simulink model "ModeAdjust"  (R2018b)
(part 6 of 35)

  PA_KeSMSw4sLyingMDSecRwRtStLgrstOtwdInwdPosMax_Val/1 -> Bus Creator74/11  "LgrstOtwdInwdPosMax"
  PA_KeSMSw4sLyingMDSecRwRtStBkReclnUpwdDnwdPosMax_Val/1 -> Bus Creator74/2  "BkReclnUpwdDnwdPosMax"
  PA_KeSMSw4sLyingMDSecRwRtStLgrstUpwdPosMin_Val/1 -> Bus Creator74/9  "LgrstUpwdPosMin"
  PA_KeSMSw4sLyingMDSecRwRtStLgrstUpwdPosMax_Val/1 -> Bus Creator74/8  "LgrstUpwdPosMax"
  PA_KeSMSw4sLyingMDSecRwRtStHdrstUpwdPosMin_Val/1 -> Bus Creator74/6  "HdrstUpwdPosMin"
  PA_KeSMSw4sLyingMDSecRwRtStFtrstUpwdDnwdPosMax_Val/1 -> Bus Creator74/14  "FtrstUpwdDnwdPosMax"
  PA_KeSMSw4sLyingMDSecRwRtStFtrstUpwdDnwdPosMin_Val/1 -> Bus Creator74/15  "FtrstUpwdDnwdPosMin"
  PA_KeSMSw4sLyingMDSecRwRtStBkReclnUpwdDnwdPos_Val/1 -> Bus Creator74/1  "BkReclnUpwdDnwdPos"
  PA_KeSMSw4sLyingMDSecRwRtStHdrstUpwdPos_Val/1 -> Bus Creator74/4  "HdrstUpwdPos"
  PA_KeSMSw4sLyingMDSecRwRtStHdrstUpwdPosMax_Val/1 -> Bus Creator74/5  "HdrstUpwdPosMax"
  PA_KeSMSw4sLyingMDSecRwRtStFtrstUpwdDnwdPos_Val/1 -> Bus Creator74/13  "FtrstUpwdDnwdPos"
  PA_KeSMSw4sRecoveryMDSecRwLtStFtrstUpwdDnwdPos_Val/1 -> Bus Creator75/13  "FtrstUpwdDnwdPos"
  PA_KeSMSw4sRecoveryMDSecRwLtStFtrstUpwdDnwdPosMin_Val/1 -> Bus Creator75/15  "FtrstUpwdDnwdPosMin"
  PA_KeSMSw4sRecoveryMDSecRwLtStFtrstUpwdDnwdPosMax_Val/1 -> Bus Creator75/14  "FtrstUpwdDnwdPosMax"
  PA_KeSMSw4sRecoveryMDSecRwLtStLgrstOtwdInwdPos_Val/1 -> Bus Creator75/10  "LgrstOtwdInwdPos"
  PA_KeSMSw4sRecoveryMDSecRwLtStLgrstOtwdInwdPosMin_Val/1 -> Bus Creator75/12  "LgrstOtwdInwdPosMin"
  PA_KeSMSw4sRecoveryMDSecRwLtStLgrstOtwdInwdPosMax_Val/1 -> Bus Creator75/11  "LgrstOtwdInwdPosMax"
  PA_KeSMSw4sRecoveryMDSecRwLtStLgrstUpwdDnwdPosMin_Val/1 -> Bus Creator75/9  "LgrstUpwdPosMin"
  PA_KeSMSw4sRecoveryMDSecRwLtStHdrstUpwdDnwdPosMax_Val/1 -> Bus Creator75/5  "HdrstUpwdPosMax"
  PA_KeSMSw4sRecoveryMDSecRwLtStBkReclnUpwdDnwdPosMax_Val/1 -> Bus Creator75/2  "BkReclnUpwdDnwdPosMax"
  PA_KeSMSw4sRecoveryMDSecRwLtStBkReclnUpwdDnwdPos_Val/1 -> Bus Creator75/1  "BkReclnUpwdDnwdPos"
  PA_KeSMSw4sRecoveryMDSecRwLtStHdrstUpwdDnwdPos_Val/1 -> Bus Creator75/4  "HdrstUpwdPos"
  PA_KeSMSw4sRecoveryMDSecRwLtStLgrstUpwdDnwdPosMax_Val/1 -> Bus Creator75/8  "LgrstUpwdPosMax"
  PA_KeSMSw4sRecoveryMDSecRwLtStLgrstUpwdDnwdPos_Val/1 -> Bus Creator75/7  "LgrstUpwdPos"
  PA_KeSMSw4sRecoveryMDSecRwLtStHdrstUpwdDnwdPosMin_Val/1 -> Bus Creator75/6  "HdrstUpwdPosMin"
  PA_KeSMSw4sRecoveryMDSecRwLtStBkReclnUpwdDnwdPosMin_Val/1 -> Bus Creator75/3  "BkReclnUpwdDnwdPosMin"
  PA_KeSMSw4sRecoveryMDSecRwRtStFtrstUpwdDnwdPos_Val/1 -> Bus Creator76/13  "FtrstUpwdDnwdPos"
  PA_KeSMSw4sRecoveryMDSecRwRtStHdrstUpwdPosMax_Val/1 -> Bus Creator76/5  "HdrstUpwdPosMax"
  PA_KeSMSw4sRecoveryMDSecRwRtStHdrstUpwdPos_Val/1 -> Bus Creator76/4  "HdrstUpwdPos"
  PA_KeSMSw4sRecoveryMDSecRwRtStBkReclnUpwdDnwdPos_Val/1 -> Bus Creator76/1  "BkReclnUpwdDnwdPos"
  PA_KeSMSw4sRecoveryMDSecRwRtStFtrstUpwdDnwdPosMin_Val/1 -> Bus Creator76/15  "FtrstUpwdDnwdPosMin"
  PA_KeSMSw4sRecoveryMDSecRwRtStFtrstUpwdDnwdPosMax_Val/1 -> Bus Creator76/14  "FtrstUpwdDnwdPosMax"
  PA_KeSMSw4sRecoveryMDSecRwRtStHdrstUpwdPosMin_Val/1 -> Bus Creator76/6  "HdrstUpwdPosMin"
  PA_KeSMSw4sRecoveryMDSecRwRtStLgrstUpwdPosMax_Val/1 -> Bus Creator76/8  "LgrstUpwdPosMax"
  PA_KeSMSw4sRecoveryMDSecRwRtStLgrstUpwdPosMin_Val/1 -> Bus Creator76/9  "LgrstUpwdPosMin"
  PA_KeSMSw4sRecoveryMDSecRwRtStBkReclnUpwdDnwdPosMax_Val/1 -> Bus Creator76/2  "BkReclnUpwdDnwdPosMax"
  PA_KeSMSw4sRecoveryMDSecRwRtStLgrstOtwdInwdPosMax_Val/1 -> Bus Creator76/11  "LgrstOtwdInwdPosMax"
  PA_KeSMSw4sRecoveryMDSecRwRtStBkReclnUpwdDnwdPosMin_Val/1 -> Bus Creator76/3  "BkReclnUpwdDnwdPosMin"
  PA_KeSMSw4sRecoveryMDSecRwRtStLgrstOtwdInwdPosMin_Val/1 -> Bus Creator76/12  "LgrstOtwdInwdPosMin"
  PA_KeSMSw4sRecoveryMDSecRwRtStLgrstOtwdInwdPos_Val/1 -> Bus Creator76/10  "LgrstOtwdInwdPos"
  PA_KeSMSw4sRecoveryMDSecRwRtStLgrstUpwdPos_Val/1 -> Bus Creator76/7  "LgrstUpwdPos"
  PA_KeSMSw4sVIPMDSecRwLtStBkReclnUpwdDnwdPosMin_Val/1 -> Bus Creator77/3  "BkReclnUpwdDnwdPosMin"
  PA_KeSMSw4sVIPMDSecRwLtStHdrstUpwdDnwdPosMin_Val/1 -> Bus Creator77/6  "HdrstUpwdPosMin"
  PA_KeSMSw4sVIPMDSecRwLtStLgrstUpwdDnwdPos_Val/1 -> Bus Creator77/7  "LgrstUpwdPos"
  PA_KeSMSw4sVIPMDSecRwLtStLgrstUpwdDnwdPosMax_Val/1 -> Bus Creator77/8  "LgrstUpwdPosMax"
  PA_KeSMSw4sVIPMDSecRwLtStHdrstUpwdDnwdPos_Val/1 -> Bus Creator77/4  "HdrstUpwdPos"
  PA_KeSMSw4sVIPMDSecRwLtStBkReclnUpwdDnwdPos_Val/1 -> Bus Creator77/1  "BkReclnUpwdDnwdPos"
  PA_KeSMSw4sVIPMDSecRwLtStBkReclnUpwdDnwdPosMax_Val/1 -> Bus Creator77/2  "BkReclnUpwdDnwdPosMax"
  PA_KeSMSw4sVIPMDSecRwLtStHdrstUpwdDnwdPosMax_Val/1 -> Bus Creator77/5  "HdrstUpwdPosMax"
  PA_KeSMSw4sVIPMDSecRwLtStLgrstUpwdDnwdPosMin_Val/1 -> Bus Creator77/9  "LgrstUpwdPosMin"
  PA_KeSMSw4sVIPMDSecRwLtStLgrstOtwdInwdPosMax_Val/1 -> Bus Creator77/11  "LgrstOtwdInwdPosMax"
  PA_KeSMSw4sVIPMDSecRwLtStLgrstOtwdInwdPosMin_Val/1 -> Bus Creator77/12  "LgrstOtwdInwdPosMin"
  PA_KeSMSw4sVIPMDSecRwLtStLgrstOtwdInwdPos_Val/1 -> Bus Creator77/10  "LgrstOtwdInwdPos"
  PA_KeSMSw4sVIPMDSecRwLtStFtrstUpwdDnwdPosMax_Val/1 -> Bus Creator77/14  "FtrstUpwdDnwdPosMax"
  PA_KeSMSw4sVIPMDSecRwLtStFtrstUpwdDnwdPosMin_Val/1 -> Bus Creator77/15  "FtrstUpwdDnwdPosMin"
  PA_KeSMSw4sVIPMDSecRwLtStFtrstUpwdDnwdPos_Val/1 -> Bus Creator77/13  "FtrstUpwdDnwdPos"
  PA_KeSMSw4sVIPMDSecRwRtStLgrstUpwdPos_Val/1 -> Bus Creator78/7  "LgrstUpwdPos"
  PA_KeSMSw4sVIPMDSecRwRtStLgrstOtwdInwdPos_Val/1 -> Bus Creator78/10  "LgrstOtwdInwdPos"
  PA_KeSMSw4sVIPMDSecRwRtStLgrstOtwdInwdPosMin_Val/1 -> Bus Creator78/12  "LgrstOtwdInwdPosMin"
  PA_KeSMSw4sVIPMDSecRwRtStBkReclnUpwdDnwdPosMin_Val/1 -> Bus Creator78/3  "BkReclnUpwdDnwdPosMin"
  PA_KeSMSw4sVIPMDSecRwRtStLgrstOtwdInwdPosMax_Val/1 -> Bus Creator78/11  "LgrstOtwdInwdPosMax"
  PA_KeSMSw4sVIPMDSecRwRtStBkReclnUpwdDnwdPosMax_Val/1 -> Bus Creator78/2  "BkReclnUpwdDnwdPosMax"
  PA_KeSMSw4sVIPMDSecRwRtStLgrstUpwdPosMin_Val/1 -> Bus Creator78/9  "LgrstUpwdPosMin"
  PA_KeSMSw4sVIPMDSecRwRtStLgrstUpwdPosMax_Val/1 -> Bus Creator78/8  "LgrstUpwdPosMax"
  PA_KeSMSw4sVIPMDSecRwRtStHdrstUpwdPosMin_Val/1 -> Bus Creator78/6  "HdrstUpwdPosMin"
  PA_KeSMSw4sVIPMDSecRwRtStFtrstUpwdDnwdPosMax_Val/1 -> Bus Creator78/14  "FtrstUpwdDnwdPosMax"
  PA_KeSMSw4sVIPMDSecRwRtStFtrstUpwdDnwdPosMin_Val/1 -> Bus Creator78/15  "FtrstUpwdDnwdPosMin"
  PA_KeSMSw4sVIPMDSecRwRtStBkReclnUpwdDnwdPos_Val/1 -> Bus Creator78/1  "BkReclnUpwdDnwdPos"
  PA_KeSMSw4sVIPMDSecRwRtStHdrstUpwdPos_Val/1 -> Bus Creator78/4  "HdrstUpwdPos"
  PA_KeSMSw4sVIPMDSecRwRtStHdrstUpwdPosMax_Val/1 -> Bus Creator78/5  "HdrstUpwdPosMax"
  PA_KeSMSw4sVIPMDSecRwRtStFtrstUpwdDnwdPos_Val/1 -> Bus Creator78/13  "FtrstUpwdDnwdPos"
  Bus Creator75/1 -> Bus Creator79/2  "RecvyLSecRwLtSt"
  Bus Creator77/1 -> Bus Creator79/3  "VipLSecRwLtSt"
  Bus Creator73/1 -> Bus Creator79/1  "LyLSecRwLtSt"
  Bus Creator76/1 -> Bus Creator80/2  "RecvyRSecRwRtSt"
  Bus Creator74/1 -> Bus Creator80/1  "LyRSecRwRtSt"
  Bus Creator78/1 -> Bus Creator80/3  "VipRSecRwRtSt"
  Bus Creator79/1 -> [Calib_2L4s]
  Bus Creator80/1 -> [Calib_2R4s]
  [Calib_2L4s] -> Bus Creator26/7  "Calib_2L4s"
  [Calib_2R4s] -> Bus Creator26/8  "Calib_2R4s"
  PA_KeSMSw6sRecoveryDrvStFtUpwdDnwdPosMax_Val/1 -> Bus Creator81/8  "FtUpwdDnwdPosMax"
  PA_KeSMSwDltTrgtPos_Val23/1 -> Bus Creator81/4  "FrwdBkwdPos"
  PA_KeSMSw6sRecoveryDrvStFtUpwdDnwdPosMin_Val/1 -> Bus Creator81/9  "FtUpwdDnwdPosMin"
  PA_KeSMSwDltTrgtPos_Val20/1 -> Bus Creator81/1  "BkReclnUpwdDnwdPos"
  PA_KeSMSwDltTrgtPos_Val22/1 -> Bus Creator81/5  "FrwdBkwdPosMax"
  PA_KeSMSwDltTrgtPos_Val19/1 -> Bus Creator81/2  "BkReclnUpwdDnwdPosMax"
  PA_KeSMSw6sRecoveryDrvStFtUpwdDnwdPos_Val/1 -> Bus Creator81/7  "FtUpwdDnwdPos"
  PA_KeSMSwDltTrgtPos_Val24/1 -> Bus Creator81/6  "FrwdBkwdPosMin"
  Bus Creator81/1 -> Bus Creator29/3  "RecvDrvSt"
  PA_KeSMSwDltTrgtPos_Val21/1 -> Bus Creator81/3  "BkReclnUpwdDnwdPosMin"
  PA_KeSMSwDltTrgtPos_Val27/1 -> Bus Creator82/3  "BkReclnUpwdDnwdPosMin"
  Bus Creator82/1 -> Bus Creator29/4  "VIPDrvSt"
  PA_KeSMSwDltTrgtPos_Val30/1 -> Bus Creator82/6  "FrwdBkwdPosMin"
  PA_KeSMSw6sVIPMDDrvStFtUpwdDnwdPos_Val/1 -> Bus Creator82/7  "FtUpwdDnwdPos"
  PA_KeSMSwDltTrgtPos_Val25/1 -> Bus Creator82/2  "BkReclnUpwdDnwdPosMax"
  PA_KeSMSwDltTrgtPos_Val28/1 -> Bus Creator82/5  "FrwdBkwdPosMax"
  PA_KeSMSwDltTrgtPos_Val26/1 -> Bus Creator82/1  "BkReclnUpwdDnwdPos"
  PA_KeSMSw6sVIPMDDrvStFtUpwdDnwdPosMin_Val/1 -> Bus Creator82/9  "FtUpwdDnwdPosMin"
  PA_KeSMSwDltTrgtPos_Val29/1 -> Bus Creator82/4  "FrwdBkwdPos"
  PA_KeSMSw6sVIPMDDrvStFtUpwdDnwdPosMax_Val/1 -> Bus Creator82/8  "FtUpwdDnwdPosMax"
  PA_KeSMSwDltTrgtPos_Val13/1 -> Bus Creator83/2  "BkReclnUpwdDnwdPosMax"
  PA_KeSMSw6sRecoveryPassStStFtUpwdDnwdPosMin_Val/1 -> Bus Creator83/9  "FtUpwdDnwdPosMin"
  PA_KeSMSw6sRecoveryPassStStFtUpwdDnwdPos_Val/1 -> Bus Creator83/7  "FtUpwdDnwdPos"
  PA_KeSMSw6sRecoveryPassStStFtUpwdDnwdPosMax_Val/1 -> Bus Creator83/8  "FtUpwdDnwdPosMax"
  PA_KeSMSwDltTrgtPos_Val15/1 -> Bus Creator83/3  "BkReclnUpwdDnwdPosMin"
  PA_KeSMSwDltTrgtPos_Val16/1 -> Bus Creator83/5  "FrwdBkwdPosMax"
  PA_KeSMSwDltTrgtPos_Val14/1 -> Bus Creator83/1  "BkReclnUpwdDnwdPos"
  PA_KeSMSwDltTrgtPos_Val18/1 -> Bus Creator83/6  "FrwdBkwdPosMin"
  PA_KeSMSwDltTrgtPos_Val17/1 -> Bus Creator83/4  "FrwdBkwdPos"
  Bus Creator83/1 -> Bus Creator32/3  "RecvPassSt"
  Bus Creator84/1 -> Bus Creator32/4  "VIPPassSt"
  PA_KeSMSwDltTrgtPos_Val35/1 -> Bus Creator84/4  "FrwdBkwdPos"
  PA_KeSMSwDltTrgtPos_Val36/1 -> Bus Creator84/6  "FrwdBkwdPosMin"
  PA_KeSMSwDltTrgtPos_Val32/1 -> Bus Creator84/1  "BkReclnUpwdDnwdPos"
  PA_KeSMSwDltTrgtPos_Val34/1 -> Bus Creator84/5  "FrwdBkwdPosMax"
  PA_KeSMSwDltTrgtPos_Val33/1 -> Bus Creator84/3  "BkReclnUpwdDnwdPosMin"
  PA_KeSMSw6sVIPMDPassStStFtUpwdDnwdPosMax_Val/1 -> Bus Creator84/8  "FtUpwdDnwdPosMax"
  PA_KeSMSw6sVIPMDPassStStFtUpwdDnwdPos_Val/1 -> Bus Creator84/7  "FtUpwdDnwdPos"
  PA_KeSMSw6sVIPMDPassStStFtUpwdDnwdPosMin_Val/1 -> Bus Creator84/9  "FtUpwdDnwdPosMin"
  PA_KeSMSwDltTrgtPos_Val31/1 -> Bus Creator84/2  "BkReclnUpwdDnwdPosMax"
  Bus Creator85/1 -> Bus Creator1/3  "RecvDrvSt"
  PA_KeSMSwDltTrgtPos_Val53/1 -> Bus Creator85/4  "FrwdBkwdPos"
  PA_KeSMSwRecoveryDrvStFtUpwdDnwdPos_Val/1 -> Bus Creator85/7  "FtUpwdDnwdPos"
  PA_KeSMSwDltTrgtPos_Val54/1 -> Bus Creator85/6  "FrwdBkwdPosMin"
  PA_KeSMSwDltTrgtPos_Val52/1 -> Bus Creator85/5  "FrwdBkwdPosMax"
  PA_KeSMSwRecoveryDrvStFtUpwdDnwdPosMin_Val/1 -> Bus Creator85/9  "FtUpwdDnwdPosMin"
  PA_KeSMSwRecoveryDrvStFtUpwdDnwdPosMax_Val/1 -> Bus Creator85/8  "FtUpwdDnwdPosMax"
  PA_KeSMSwDltTrgtPos_Val50/1 -> Bus Creator85/1  "BkReclnUpwdDnwdPos"
  PA_KeSMSwDltTrgtPos_Val51/1 -> Bus Creator85/3  "BkReclnUpwdDnwdPosMin"
  PA_KeSMSwDltTrgtPos_Val49/1 -> Bus Creator85/2  "BkReclnUpwdDnwdPosMax"
  PA_KeSMSwDltTrgtPos_Val55/1 -> Bus Creator86/2  "BkReclnUpwdDnwdPosMax"
  PA_KeSMSwDltTrgtPos_Val57/1 -> Bus Creator86/3  "BkReclnUpwdDnwdPosMin"
  PA_KeSMSwDltTrgtPos_Val56/1 -> Bus Creator86/1  "BkReclnUpwdDnwdPos"
  PA_KeSMSwVIPMDDrvStFtUpwdDnwdPosMax_Val/1 -> Bus Creator86/8  "FtUpwdDnwdPosMax"
  PA_KeSMSwVIPMDDrvStFtUpwdDnwdPosMin_Val/1 -> Bus Creator86/9  "FtUpwdDnwdPosMin"
  PA_KeSMSwDltTrgtPos_Val58/1 -> Bus Creator86/5  "FrwdBkwdPosMax"
  PA_KeSMSwDltTrgtPos_Val60/1 -> Bus Creator86/6  "FrwdBkwdPosMin"
  PA_KeSMSwVIPMDDrvStFtUpwdDnwdPos_Val/1 -> Bus Creator86/7  "FtUpwdDnwdPos"
  PA_KeSMSwDltTrgtPos_Val59/1 -> Bus Creator86/4  "FrwdBkwdPos"
  Bus Creator86/1 -> Bus Creator1/4  "VIPDrvSt"
  Bus Creator87/1 -> Bus Creator5/3  "RecvPassSt"
  Bus Creator88/1 -> Bus Creator5/4  "VIPPassSt"
  PA_KeSMSwDltTrgtPos_Val47/1 -> Bus Creator88/4  "FrwdBkwdPos"
  PA_KeSMSwVIPMDPassStStFtUpwdDnwdPos_Val/1 -> Bus Creator88/7  "FtUpwdDnwdPos"
  PA_KeSMSwDltTrgtPos_Val48/1 -> Bus Creator88/6  "FrwdBkwdPosMin"
  PA_KeSMSwDltTrgtPos_Val46/1 -> Bus Creator88/5  "FrwdBkwdPosMax"
  PA_KeSMSwVIPMDPassStStFtUpwdDnwdPosMin_Val/1 -> Bus Creator88/9  "FtUpwdDnwdPosMin"
  PA_KeSMSwVIPMDPassStStFtUpwdDnwdPosMax_Val/1 -> Bus Creator88/8  "FtUpwdDnwdPosMax"
  PA_KeSMSwDltTrgtPos_Val44/1 -> Bus Creator88/1  "BkReclnUpwdDnwdPos"
  PA_KeSMSwDltTrgtPos_Val45/1 -> Bus Creator88/3  "BkReclnUpwdDnwdPosMin"
  PA_KeSMSwDltTrgtPos_Val43/1 -> Bus Creator88/2  "BkReclnUpwdDnwdPosMax"
  PA_KeSMSwDltTrgtPos_Val41/1 -> Bus Creator87/4  "FrwdBkwdPos"
  PA_KeSMSwRecoveryPassStStFtUpwdDnwdPos_Val/1 -> Bus Creator87/7  "FtUpwdDnwdPos"
  PA_KeSMSwDltTrgtPos_Val42/1 -> Bus Creator87/6  "FrwdBkwdPosMin"
  PA_KeSMSwDltTrgtPos_Val40/1 -> Bus Creator87/5  "FrwdBkwdPosMax"
  PA_KeSMSwRecoveryPassStStFtUpwdDnwdPosMin_Val/1 -> Bus Creator87/9  "FtUpwdDnwdPosMin"
  PA_KeSMSwRecoveryPassStStFtUpwdDnwdPosMax_Val/1 -> Bus Creator87/8  "FtUpwdDnwdPosMax"
  PA_KeSMSwDltTrgtPos_Val38/1 -> Bus Creator87/1  "BkReclnUpwdDnwdPos"
  PA_KeSMSwDltTrgtPos_Val37/1 -> Bus Creator87/2  "BkReclnUpwdDnwdPosMax"
  PA_KeSMSwDltTrgtPos_Val39/1 -> Bus Creator87/3  "BkReclnUpwdDnwdPosMin"
  PA_KeSMSwDltTrgtPos_Val84/1 -> Bus Creator89/7  "FrwdBkwdPos"
  PA_KeSMSwDltTrgtPos_Val65/1 -> Bus Creator89/4  "BkReclnUpwdDnwdPos"
  PA_KeSMSwDltTrgtPos_Val64/1 -> Bus Creator89/5  "BkReclnUpwdDnwdPosMax"
  PA_KeSMSwDltTrgtPos_Val72/1 -> Bus Creator89/12  "HdrstUpwdPosMin"
  PA_KeSMSwDltTrgtPos_Val82/1 -> Bus Creator89/8  "FrwdBkwdPosMax"
  PA_KeSMSw6sIntimacyMdSecRwLtStLtwdRtwdPosMin_Val/1 -> Bus Creator89/18  "LtwdRtwdPosMin"
  PA_KeSMSwDltTrgtPos_Val75/1 -> Bus Creator89/15  "LgrstUpwdPosMin"
  PA_KeSMSwDltTrgtPos_Val62/1 -> Bus Creator89/1  "ArmScrnPos"
  PA_KeSMSwDltTrgtPos_Val83/1 -> Bus Creator89/9  "FrwdBkwdPosMin"
  Bus Creator89/1 -> Bus Creator37/5  "INTMSecRwLtSt"
  PA_KeSMSw6sIntimacyMdSecRwLtStLtwdRtwdPos_Val/1 -> Bus Creator89/16  "LtwdRtwdPos"
  PA_KeSMSwDltTrgtPos_Val74/1 -> Bus Creator89/13  "LgrstUpwdPos"
  PA_KeSMSwDltTrgtPos_Val63/1 -> Bus Creator89/3  "ArmScrnPosMin"
  PA_KeSMSwDltTrgtPos_Val70/1 -> Bus Creator89/11  "HdrstUpwdPosMax"
  PA_KeSMSw6sIntimacyMdSecRwLtStLtwdRtwdPosMax_Val/1 -> Bus Creator89/17  "LtwdRtwdPosMax"
  PA_KeSMSwDltTrgtPos_Val61/1 -> Bus Creator89/2  "ArmScrnPosMax"
  PA_KeSMSwDltTrgtPos_Val71/1 -> Bus Creator89/10  "HdrstUpwdPos"
  PA_KeSMSwDltTrgtPos_Val66/1 -> Bus Creator89/6  "BkReclnUpwdDnwdPosMin"
  PA_KeSMSwDltTrgtPos_Val73/1 -> Bus Creator89/14  "LgrstUpwdPosMax"
  PA_KeSMSwDltTrgtPos_Val68/1 -> Bus Creator90/9  "FrwdBkwdPosMin"
  PA_KeSMSwDltTrgtPos_Val87/1 -> Bus Creator90/12  "HdrstUpwdPosMin"
  PA_KeSMSwDltTrgtPos_Val67/1 -> Bus Creator90/7  "FrwdBkwdPos"
  PA_KeSMSw6sIntimacyMdSecRwRtStLtwdRtwdPos_Val/1 -> Bus Creator90/16  "LtwdRtwdPos"
  PA_KeSMSwDltTrgtPos_Val69/1 -> Bus Creator90/8  "FrwdBkwdPosMax"
  PA_KeSMSw6sIntimacyMdSecRwRtStLtwdRtwdPosMax_Val/1 -> Bus Creator90/17  "LtwdRtwdPosMax"
  PA_KeSMSwDltTrgtPos_Val76/1 -> Bus Creator90/2  "ArmScrnPosMax"
  PA_KeSMSwDltTrgtPos_Val78/1 -> Bus Creator90/3  "ArmScrnPosMin"
  PA_KeSMSwDltTrgtPos_Val81/1 -> Bus Creator90/6  "BkReclnUpwdDnwdPosMin"
  PA_KeSMSw6sIntimacyMdSecRwRtStLtwdRtwdPosMin_Val/1 -> Bus Creator90/18  "LtwdRtwdPosMin"
  PA_KeSMSwDltTrgtPos_Val86/1 -> Bus Creator90/10  "HdrstUpwdPos"
  PA_KeSMSwDltTrgtPos_Val80/1 -> Bus Creator90/4  "BkReclnUpwdDnwdPos"
  Bus Creator90/1 -> Bus Creator42/5  "INTMSecRwRtSt"
  PA_KeSMSwDltTrgtPos_Val90/1 -> Bus Creator90/15  "LgrstUpwdPosMin"
  PA_KeSMSwDltTrgtPos_Val89/1 -> Bus Creator90/13  "LgrstUpwdPos"
  PA_KeSMSwDltTrgtPos_Val77/1 -> Bus Creator90/1  "ArmScrnPos"
  PA_KeSMSwDltTrgtPos_Val79/1 -> Bus Creator90/5  "BkReclnUpwdDnwdPosMax"
  PA_KeSMSwDltTrgtPos_Val88/1 -> Bus Creator90/14  "LgrstUpwdPosMax"
  PA_KeSMSwDltTrgtPos_Val85/1 -> Bus Creator90/11  "HdrstUpwdPosMax"
  PA_KeSMSwDltTrgtPos_Val290/1 -> Bus Creator91/8  "FrwdBkwdPosMax"
  PA_KeSMSwDltTrgtPos_Val100/1 -> Bus Creator91/11  "HdrstUpwdPosMax"
  PA_KeSMSwDltTrgtPos_Val289/1 -> Bus Creator91/7  "FrwdBkwdPos"
  PA_KeSMSwDltTrgtPos_Val96/1 -> Bus Creator91/6  "BkReclnUpwdDnwdPosMin"
  PA_KeSMSwDltTrgtPos_Val92/1 -> Bus Creator91/1  "ArmScrnPos"
  PA_KeSMSwDltTrgtPos_Val291/1 -> Bus Creator91/9  "FrwdBkwdPosMin"
  PA_KeSMSwDltTrgtPos_Val95/1 -> Bus Creator91/4  "BkReclnUpwdDnwdPos"
  PA_KeSMSwDltTrgtPos_Val103/1 -> Bus Creator91/14  "LgrstUpwdPosMax"
  PA_KeSMSwDltTrgtPos_Val105/1 -> Bus Creator91/15  "LgrstUpwdPosMin"
  PA_KeSMSwDltTrgtPos_Val94/1 -> Bus Creator91/5  "BkReclnUpwdDnwdPosMax"
  PA_KeSMSwDltTrgtPos_Val104/1 -> Bus Creator91/13  "LgrstUpwdPos"
  PA_KeSMSwDltTrgtPos_Val101/1 -> Bus Creator91/10  "HdrstUpwdPos"
  Bus Creator91/1 -> Bus Creator14/5  "INTMSecRwLtSt"
  PA_KeSMSwIntimacyMdSecRwLtStLtwdRtwdPosMax_Val/1 -> Bus Creator91/17  "LtwdRtwdPosMax"
  PA_KeSMSwIntimacyMdSecRwLtStLtwdRtwdPosMin_Val/1 -> Bus Creator91/18  "LtwdRtwdPosMin"
  PA_KeSMSwIntimacyMdSecRwLtStLtwdRtwdPos_Val/1 -> Bus Creator91/16  "LtwdRtwdPos"
  PA_KeSMSwDltTrgtPos_Val93/1 -> Bus Creator91/3  "ArmScrnPosMin"
  PA_KeSMSwDltTrgtPos_Val102/1 -> Bus Creator91/12  "HdrstUpwdPosMin"
  PA_KeSMSwDltTrgtPos_Val91/1 -> Bus Creator91/2  "ArmScrnPosMax"
  PA_KeSMSwDltTrgtPos_Val293/1 -> Bus Creator92/8  "FrwdBkwdPosMax"
  PA_KeSMSwDltTrgtPos_Val115/1 -> Bus Creator92/11  "HdrstUpwdPosMax"
  PA_KeSMSwDltTrgtPos_Val294/1 -> Bus Creator92/7  "FrwdBkwdPos"
  PA_KeSMSwDltTrgtPos_Val111/1 -> Bus Creator92/6  "BkReclnUpwdDnwdPosMin"
  PA_KeSMSwDltTrgtPos_Val107/1 -> Bus Creator92/1  "ArmScrnPos"
  PA_KeSMSwDltTrgtPos_Val292/1 -> Bus Creator92/9  "FrwdBkwdPosMin"
  PA_KeSMSwDltTrgtPos_Val110/1 -> Bus Creator92/4  "BkReclnUpwdDnwdPos"
  PA_KeSMSwDltTrgtPos_Val118/1 -> Bus Creator92/14  "LgrstUpwdPosMax"
  PA_KeSMSwDltTrgtPos_Val120/1 -> Bus Creator92/15  "LgrstUpwdPosMin"
  PA_KeSMSwDltTrgtPos_Val109/1 -> Bus Creator92/5  "BkReclnUpwdDnwdPosMax"
  PA_KeSMSwDltTrgtPos_Val119/1 -> Bus Creator92/13  "LgrstUpwdPos"
  PA_KeSMSwDltTrgtPos_Val116/1 -> Bus Creator92/10  "HdrstUpwdPos"
  Bus Creator92/1 -> Bus Creator15/5  "INTMSecRwRtSt"
  PA_KeSMSwIntimacyMdSecRwRtStLtwdRtwdPosMax_Val/1 -> Bus Creator92/17  "LtwdRtwdPosMax"
  PA_KeSMSwIntimacyMdSecRwRtStLtwdRtwdPosMin_Val/1 -> Bus Creator92/18  "LtwdRtwdPosMin"
  PA_KeSMSwIntimacyMdSecRwRtStLtwdRtwdPos_Val/1 -> Bus Creator92/16  "LtwdRtwdPos"
  PA_KeSMSwDltTrgtPos_Val108/1 -> Bus Creator92/3  "ArmScrnPosMin"
  PA_KeSMSwDltTrgtPos_Val117/1 -> Bus Creator92/12  "HdrstUpwdPosMin"
  PA_KeSMSwDltTrgtPos_Val106/1 -> Bus Creator92/2  "ArmScrnPosMax"
  PA_KeSMSw6sFamilyMdSecRwLtStFrwdBkwdPosMin_Val/1 -> Bus Creator93/9  "FrwdBkwdPosMin"
  PA_KeSMSwDltTrgtPos_Val129/1 -> Bus Creator93/12  "HdrstUpwdPosMin"
  PA_KeSMSw6sFamilyMdSecRwLtStFrwdBkwdPos_Val/1 -> Bus Creator93/7  "FrwdBkwdPos"
  PA_KeSMSw6sFamilyMdSecRwLtStLtwdRtwdPos_Val/1 -> Bus Creator93/16  "LtwdRtwdPos"
  PA_KeSMSw6sFamilyMdSecRwLtStFrwdBkwdPosMax_Val/1 -> Bus Creator93/8  "FrwdBkwdPosMax"
  PA_KeSMSw6sFamilyMdSecRwLtStLtwdRtwdPosMax_Val/1 -> Bus Creator93/17  "LtwdRtwdPosMax"
  PA_KeSMSwDltTrgtPos_Val121/1 -> Bus Creator93/2  "ArmScrnPosMax"
  PA_KeSMSwDltTrgtPos_Val123/1 -> Bus Creator93/3  "ArmScrnPosMin"
  PA_KeSMSwDltTrgtPos_Val126/1 -> Bus Creator93/6  "BkReclnUpwdDnwdPosMin"
  PA_KeSMSw6sFamilyMdSecRwLtStLtwdRtwdPosMin_Val/1 -> Bus Creator93/18  "LtwdRtwdPosMin"
  PA_KeSMSwDltTrgtPos_Val128/1 -> Bus Creator93/10  "HdrstUpwdPos"
  PA_KeSMSwDltTrgtPos_Val125/1 -> Bus Creator93/4  "BkReclnUpwdDnwdPos"
  Bus Creator93/1 -> Bus Creator37/6  "FamlyLSecRwLtSt"
  PA_KeSMSwDltTrgtPos_Val132/1 -> Bus Creator93/15  "LgrstUpwdPosMin"
  PA_KeSMSwDltTrgtPos_Val131/1 -> Bus Creator93/13  "LgrstUpwdPos"
  PA_KeSMSwDltTrgtPos_Val122/1 -> Bus Creator93/1  "ArmScrnPos"
  PA_KeSMSwDltTrgtPos_Val124/1 -> Bus Creator93/5  "BkReclnUpwdDnwdPosMax"
  PA_KeSMSwDltTrgtPos_Val130/1 -> Bus Creator93/14  "LgrstUpwdPosMax"
  PA_KeSMSwDltTrgtPos_Val127/1 -> Bus Creator93/11  "HdrstUpwdPosMax"
  PA_KeSMSw6sFamilyRMdSecRwLtStFrwdBkwdPosMin_Val/1 -> Bus Creator94/9  "FrwdBkwdPosMin"
  PA_KeSMSwDltTrgtPos_Val201/1 -> Bus Creator94/12  "HdrstUpwdPosMin"
  PA_KeSMSw6sFamilyRMdSecRwLtStFrwdBkwdPos_Val/1 -> Bus Creator94/7  "FrwdBkwdPos"
  PA_KeSMSw6sFamilyRMdSecRwLtStLtwdRtwdPos_Val/1 -> Bus Creator94/16  "LtwdRtwdPos"
  PA_KeSMSw6sFamilyRMdSecRwLtStFrwdBkwdPosMax_Val/1 -> Bus Creator94/8  "FrwdBkwdPosMax"
  PA_KeSMSw6sFamilyRMdSecRwLtStLtwdRtwdPosMax_Val/1 -> Bus Creator94/17  "LtwdRtwdPosMax"
  PA_KeSMSwDltTrgtPos_Val193/1 -> Bus Creator94/2  "ArmScrnPosMax"
  PA_KeSMSwDltTrgtPos_Val195/1 -> Bus Creator94/3  "ArmScrnPosMin"
  PA_KeSMSwDltTrgtPos_Val198/1 -> Bus Creator94/6  "BkReclnUpwdDnwdPosMin"
  PA_KeSMSw6sFamilyRMdSecRwLtStLtwdRtwdPosMin_Val/1 -> Bus Creator94/18  "LtwdRtwdPosMin"
  PA_KeSMSwDltTrgtPos_Val200/1 -> Bus Creator94/10  "HdrstUpwdPos"
  PA_KeSMSwDltTrgtPos_Val197/1 -> Bus Creator94/4  "BkReclnUpwdDnwdPos"
  Bus Creator94/1 -> Bus Creator37/7  "FamlyRSecRwLtSt"
  PA_KeSMSwDltTrgtPos_Val204/1 -> Bus Creator94/15  "LgrstUpwdPosMin"
  PA_KeSMSwDltTrgtPos_Val203/1 -> Bus Creator94/13  "LgrstUpwdPos"
  PA_KeSMSwDltTrgtPos_Val194/1 -> Bus Creator94/1  "ArmScrnPos"
  PA_KeSMSwDltTrgtPos_Val196/1 -> Bus Creator94/5  "BkReclnUpwdDnwdPosMax"
  PA_KeSMSwDltTrgtPos_Val202/1 -> Bus Creator94/14  "LgrstUpwdPosMax"
  PA_KeSMSwDltTrgtPos_Val199/1 -> Bus Creator94/11  "HdrstUpwdPosMax"
  PA_KeSMSw6sFamilyMdSecRwRtStFrwdBkwdPosMin_Val/1 -> Bus Creator95/9  "FrwdBkwdPosMin"
  PA_KeSMSwDltTrgtPos_Val141/1 -> Bus Creator95/12  "HdrstUpwdPosMin"
  PA_KeSMSw6sFamilyMdSecRwRtStFrwdBkwdPos_Val/1 -> Bus Creator95/7  "FrwdBkwdPos"
  PA_KeSMSw6sFamilyMdSecRwRtStLtwdRtwdPos_Val/1 -> Bus Creator95/16  "LtwdRtwdPos"
  PA_KeSMSw6sFamilyMdSecRwRtStFrwdBkwdPosMax_Val/1 -> Bus Creator95/8  "FrwdBkwdPosMax"
  PA_KeSMSw6sFamilyMdSecRwRtStLtwdRtwdPosMax_Val/1 -> Bus Creator95/17  "LtwdRtwdPosMax"
  PA_KeSMSwDltTrgtPos_Val133/1 -> Bus Creator95/2  "ArmScrnPosMax"
  PA_KeSMSwDltTrgtPos_Val135/1 -> Bus Creator95/3  "ArmScrnPosMin"
  PA_KeSMSwDltTrgtPos_Val138/1 -> Bus Creator95/6  "BkReclnUpwdDnwdPosMin"
  PA_KeSMSw6sFamilyMdSecRwRtStLtwdRtwdPosMin_Val/1 -> Bus Creator95/18  "LtwdRtwdPosMin"
  PA_KeSMSwDltTrgtPos_Val140/1 -> Bus Creator95/10  "HdrstUpwdPos"
  PA_KeSMSwDltTrgtPos_Val137/1 -> Bus Creator95/4  "BkReclnUpwdDnwdPos"
  Bus Creator95/1 -> Bus Creator42/6  "FamlyLSecRwRtSt"
  PA_KeSMSwDltTrgtPos_Val144/1 -> Bus Creator95/15  "LgrstUpwdPosMin"
  PA_KeSMSwDltTrgtPos_Val143/1 -> Bus Creator95/13  "LgrstUpwdPos"
  PA_KeSMSwDltTrgtPos_Val134/1 -> Bus Creator95/1  "ArmScrnPos"
  PA_KeSMSwDltTrgtPos_Val136/1 -> Bus Creator95/5  "BkReclnUpwdDnwdPosMax"
  PA_KeSMSwDltTrgtPos_Val142/1 -> Bus Creator95/14  "LgrstUpwdPosMax"
  PA_KeSMSwDltTrgtPos_Val139/1 -> Bus Creator95/11  "HdrstUpwdPosMax"
  PA_KeSMSw6sFamilyRMdSecRwRtStFrwdBkwdPosMin_Val/1 -> Bus Creator96/9  "FrwdBkwdPosMin"
  PA_KeSMSwDltTrgtPos_Val213/1 -> Bus Creator96/12  "HdrstUpwdPosMin"
  PA_KeSMSw6sFamilyRMdSecRwRtStFrwdBkwdPos_Val/1 -> Bus Creator96/7  "FrwdBkwdPos"
  PA_KeSMSw6sFamilyRMdSecRwRtStLtwdRtwdPos_Val/1 -> Bus Creator96/16  "LtwdRtwdPos"
  PA_KeSMSw6sFamilyRMdSecRwRtStFrwdBkwdPosMax_Val/1 -> Bus Creator96/8  "FrwdBkwdPosMax"
  PA_KeSMSw6sFamilyRMdSecRwRtStLtwdRtwdPosMax_Val/1 -> Bus Creator96/17  "LtwdRtwdPosMax"
  PA_KeSMSwDltTrgtPos_Val205/1 -> Bus Creator96/2  "ArmScrnPosMax"
  PA_KeSMSwDltTrgtPos_Val207/1 -> Bus Creator96/3  "ArmScrnPosMin"
  PA_KeSMSwDltTrgtPos_Val210/1 -> Bus Creator96/6  "BkReclnUpwdDnwdPosMin"
  PA_KeSMSw6sFamilyRMdSecRwRtStLtwdRtwdPosMin_Val/1 -> Bus Creator96/18  "LtwdRtwdPosMin"
  PA_KeSMSwDltTrgtPos_Val212/1 -> Bus Creator96/10  "HdrstUpwdPos"
  PA_KeSMSwDltTrgtPos_Val209/1 -> Bus Creator96/4  "BkReclnUpwdDnwdPos"
  Bus Creator96/1 -> Bus Creator42/7  "FamlyRSecRwRtSt"
  PA_KeSMSwDltTrgtPos_Val216/1 -> Bus Creator96/15  "LgrstUpwdPosMin"
  PA_KeSMSwDltTrgtPos_Val215/1 -> Bus Creator96/13  "LgrstUpwdPos"
  PA_KeSMSwDltTrgtPos_Val206/1 -> Bus Creator96/1  "ArmScrnPos"
  PA_KeSMSwDltTrgtPos_Val208/1 -> Bus Creator96/5  "BkReclnUpwdDnwdPosMax"
  PA_KeSMSwDltTrgtPos_Val214/1 -> Bus Creator96/14  "LgrstUpwdPosMax"
  PA_KeSMSwDltTrgtPos_Val211/1 -> Bus Creator96/11  "HdrstUpwdPosMax"
  PA_KeSMSwDltTrgtPos_Val225/1 -> Bus Creator98/12  "HdrstUpwdPosMin"
  PA_KeSMSwFamilyRMdSecRwLtStFrwdBkwdPosMax_Val/1 -> Bus Creator98/8  "FrwdBkwdPosMax"
  PA_KeSMSwFamilyRMdSecRwLtStLtwdRtwdPos_Val/1 -> Bus Creator98/16  "LtwdRtwdPos"
  Bus Creator97/1 -> Bus Creator14/6  "FamlyLSecRwLtSt"
  PA_KeSMSwFamilyMdSecRwLtStFrwdBkwdPosMin_Val/1 -> Bus Creator97/9  "FrwdBkwdPosMin"
  PA_KeSMSwFamilyRMdSecRwLtStFrwdBkwdPos_Val/1 -> Bus Creator98/7  "FrwdBkwdPos"
  PA_KeSMSwDltTrgtPos_Val228/1 -> Bus Creator98/15  "LgrstUpwdPosMin"
  PA_KeSMSwDltTrgtPos_Val222/1 -> Bus Creator98/6  "BkReclnUpwdDnwdPosMin"
  PA_KeSMSwFamilyRMdSecRwLtStLtwdRtwdPosMin_Val/1 -> Bus Creator98/18  "LtwdRtwdPosMin"
  PA_KeSMSwDltTrgtPos_Val227/1 -> Bus Creator98/13  "LgrstUpwdPos"
  PA_KeSMSwFamilyRMdSecRwLtStLtwdRtwdPosMax_Val/1 -> Bus Creator98/17  "LtwdRtwdPosMax"
  PA_KeSMSwDltTrgtPos_Val220/1 -> Bus Creator98/5  "BkReclnUpwdDnwdPosMax"
  Bus Creator98/1 -> Bus Creator14/7  "FamlyRSecRwLtSt"
  PA_KeSMSwDltTrgtPos_Val219/1 -> Bus Creator98/3  "ArmScrnPosMin"
  PA_KeSMSwDltTrgtPos_Val162/1 -> Bus Creator97/6  "BkReclnUpwdDnwdPosMin"
  PA_KeSMSwDltTrgtPos_Val158/1 -> Bus Creator97/1  "ArmScrnPos"
  PA_KeSMSwFamilyRMdSecRwLtStFrwdBkwdPosMin_Val/1 -> Bus Creator98/9  "FrwdBkwdPosMin"
  PA_KeSMSwDltTrgtPos_Val161/1 -> Bus Creator97/4  "BkReclnUpwdDnwdPos"
  PA_KeSMSwDltTrgtPos_Val168/1 -> Bus Creator97/15  "LgrstUpwdPosMin"
  PA_KeSMSwFamilyMdSecRwLtStFrwdBkwdPosMax_Val/1 -> Bus Creator97/8  "FrwdBkwdPosMax"
  PA_KeSMSwDltTrgtPos_Val163/1 -> Bus Creator97/11  "HdrstUpwdPosMax"
  PA_KeSMSwDltTrgtPos_Val218/1 -> Bus Creator98/1  "ArmScrnPos"
  PA_KeSMSwDltTrgtPos_Val224/1 -> Bus Creator98/10  "HdrstUpwdPos"
  PA_KeSMSwDltTrgtPos_Val159/1 -> Bus Creator97/3  "ArmScrnPosMin"
  PA_KeSMSwDltTrgtPos_Val164/1 -> Bus Creator97/10  "HdrstUpwdPos"
  PA_KeSMSwDltTrgtPos_Val223/1 -> Bus Creator98/11  "HdrstUpwdPosMax"
  PA_KeSMSwFamilyMdSecRwLtStLtwdRtwdPosMin_Val/1 -> Bus Creator97/18  "LtwdRtwdPosMin"
  PA_KeSMSwDltTrgtPos_Val167/1 -> Bus Creator97/13  "LgrstUpwdPos"
  PA_KeSMSwFamilyMdSecRwLtStLtwdRtwdPosMax_Val/1 -> Bus Creator97/17  "LtwdRtwdPosMax"
  PA_KeSMSwDltTrgtPos_Val157/1 -> Bus Creator97/2  "ArmScrnPosMax"
  PA_KeSMSwDltTrgtPos_Val166/1 -> Bus Creator97/14  "LgrstUpwdPosMax"
  PA_KeSMSwDltTrgtPos_Val217/1 -> Bus Creator98/2  "ArmScrnPosMax"
  PA_KeSMSwFamilyMdSecRwLtStLtwdRtwdPos_Val/1 -> Bus Creator97/16  "LtwdRtwdPos"
  PA_KeSMSwDltTrgtPos_Val165/1 -> Bus Creator97/12  "HdrstUpwdPosMin"
  PA_KeSMSwFamilyMdSecRwLtStFrwdBkwdPos_Val/1 -> Bus Creator97/7  "FrwdBkwdPos"
  PA_KeSMSwDltTrgtPos_Val226/1 -> Bus Creator98/14  "LgrstUpwdPosMax"
  PA_KeSMSwDltTrgtPos_Val160/1 -> Bus Creator97/5  "BkReclnUpwdDnwdPosMax"
  PA_KeSMSwDltTrgtPos_Val221/1 -> Bus Creator98/4  "BkReclnUpwdDnwdPos"
  PA_KeSMSwDltTrgtPos_Val232/1 -> Bus Creator100/5  "BkReclnUpwdDnwdPosMax"
  PA_KeSMSwDltTrgtPos_Val235/1 -> Bus Creator100/11  "HdrstUpwdPosMax"
  PA_KeSMSwDltTrgtPos_Val238/1 -> Bus Creator100/14  "LgrstUpwdPosMax"
  PA_KeSMSwDltTrgtPos_Val230/1 -> Bus Creator100/1  "ArmScrnPos"
  PA_KeSMSwFamilyRMdSecRwRtStLtwdRtwdPos_Val/1 -> Bus Creator100/16  "LtwdRtwdPos"
  PA_KeSMSwDltTrgtPos_Val236/1 -> Bus Creator100/10  "HdrstUpwdPos"
  PA_KeSMSwDltTrgtPos_Val231/1 -> Bus Creator100/3  "ArmScrnPosMin"
  PA_KeSMSwFamilyRMdSecRwRtStFrwdBkwdPos_Val/1 -> Bus Creator100/7  "FrwdBkwdPos"
  PA_KeSMSwFamilyRMdSecRwRtStFrwdBkwdPosMax_Val/1 -> Bus Creator100/8  "FrwdBkwdPosMax"
  Bus Creator100/1 -> Bus Creator15/7  "FamlyRSecRwRtSt"
  PA_KeSMSwFamilyRMdSecRwRtStLtwdRtwdPosMin_Val/1 -> Bus Creator100/18  "LtwdRtwdPosMin"
  PA_KeSMSwFamilyRMdSecRwRtStFrwdBkwdPosMin_Val/1 -> Bus Creator100/9  "FrwdBkwdPosMin"
  Bus Creator99/1 -> Bus Creator15/6  "FamlyLSecRwRtSt"
  PA_KeSMSwDltTrgtPos_Val237/1 -> Bus Creator100/12  "HdrstUpwdPosMin"
  PA_KeSMSwDltTrgtPos_Val229/1 -> Bus Creator100/2  "ArmScrnPosMax"
  PA_KeSMSwDltTrgtPos_Val234/1 -> Bus Creator100/6  "BkReclnUpwdDnwdPosMin"
  PA_KeSMSwFamilyMdSecRwRtStFrwdBkwdPos_Val/1 -> Bus Creator99/7  "FrwdBkwdPos"
  PA_KeSMSwDltTrgtPos_Val173/1 -> Bus Creator99/4  "BkReclnUpwdDnwdPos"
  PA_KeSMSwDltTrgtPos_Val171/1 -> Bus Creator99/3  "ArmScrnPosMin"
  PA_KeSMSwDltTrgtPos_Val233/1 -> Bus Creator100/4  "BkReclnUpwdDnwdPos"
  PA_KeSMSwDltTrgtPos_Val178/1 -> Bus Creator99/14  "LgrstUpwdPosMax"
  PA_KeSMSwFamilyMdSecRwRtStFrwdBkwdPosMin_Val/1 -> Bus Creator99/9  "FrwdBkwdPosMin"
  PA_KeSMSwFamilyRMdSecRwRtStLtwdRtwdPosMax_Val/1 -> Bus Creator100/17  "LtwdRtwdPosMax"
  PA_KeSMSwFamilyMdSecRwRtStLtwdRtwdPosMin_Val/1 -> Bus Creator99/18  "LtwdRtwdPosMin"
  PA_KeSMSwDltTrgtPos_Val240/1 -> Bus Creator100/15  "LgrstUpwdPosMin"
  PA_KeSMSwFamilyMdSecRwRtStLtwdRtwdPos_Val/1 -> Bus Creator99/16  "LtwdRtwdPos"
  PA_KeSMSwDltTrgtPos_Val175/1 -> Bus Creator99/11  "HdrstUpwdPosMax"
  PA_KeSMSwDltTrgtPos_Val170/1 -> Bus Creator99/1  "ArmScrnPos"
  PA_KeSMSwDltTrgtPos_Val180/1 -> Bus Creator99/15  "LgrstUpwdPosMin"
  PA_KeSMSwDltTrgtPos_Val172/1 -> Bus Creator99/5  "BkReclnUpwdDnwdPosMax"
  PA_KeSMSwFamilyMdSecRwRtStLtwdRtwdPosMax_Val/1 -> Bus Creator99/17  "LtwdRtwdPosMax"
  PA_KeSMSwDltTrgtPos_Val176/1 -> Bus Creator99/10  "HdrstUpwdPos"
  PA_KeSMSwDltTrgtPos_Val174/1 -> Bus Creator99/6  "BkReclnUpwdDnwdPosMin"
  PA_KeSMSwDltTrgtPos_Val179/1 -> Bus Creator99/13  "LgrstUpwdPos"
  PA_KeSMSwFamilyMdSecRwRtStFrwdBkwdPosMax_Val/1 -> Bus Creator99/8  "FrwdBkwdPosMax"
  PA_KeSMSwDltTrgtPos_Val239/1 -> Bus Creator100/13  "LgrstUpwdPos"
  PA_KeSMSwDltTrgtPos_Val169/1 -> Bus Creator99/2  "ArmScrnPosMax"
  PA_KeSMSwDltTrgtPos_Val177/1 -> Bus Creator99/12  "HdrstUpwdPosMin"
  PA_KeSMSw4sLyingMDSecRwLtStHdrstFrwdBkwdnwdPos_Val/1 -> Bus Creator73/16  "HdrstFrwdBkwdnwdPos"
  PA_KeSMSw4sLyingMDSecRwLtStHdrstFrwdBkwdnwdPosMax_Val/1 -> Bus Creator73/17  "HdrstFrwdBkwdnwdPosMax"
  PA_KeSMSw4sLyingMDSecRwLtStHdrstFrwdBkwdnwdPosMin_Val/1 -> Bus Creator73/18  "HdrstFrwdBkwdnwdPosMin"
  PA_KeSMSw4sRecoveryMDSecRwLtStHdrstFrwdBkwdPos_Val/1 -> Bus Creator75/16  "HdrstFrwdBkwdnwdPos"
  PA_KeSMSw4sRecoveryMDSecRwLtStHdrstFrwdBkwdPosMax_Val/1 -> Bus Creator75/17  "HdrstFrwdBkwdnwdPosMax"
  PA_KeSMSw4sRecoveryMDSecRwLtStHdrstFrwdBkwdPosMin_Val/1 -> Bus Creator75/18  "HdrstFrwdBkwdnwdPosMin"
  PA_KeSMSw4sVIPMDSecRwLtStHdrstFrwdBkwdPos_Val/1 -> Bus Creator77/16  "HdrstFrwdBkwdnwdPos"
  PA_KeSMSw4sVIPMDSecRwLtStHdrstFrwdBkwdPosMax_Val/1 -> Bus Creator77/17  "HdrstFrwdBkwdnwdPosMax"
  PA_KeSMSw4sVIPMDSecRwLtStHdrstFrwdBkwdPosMin_Val/1 -> Bus Creator77/18  "HdrstFrwdBkwdnwdPosMin"
  PA_KeSMSw4sLyingMDSecRwRtStHdrstFrwdBkwdnwdPos_Val/1 -> Bus Creator74/16  "HdrstFrwdBkwdnwdPos"
  PA_KeSMSw4sLyingMDSecRwRtStHdrstFrwdBkwdnwdPosMax_Val/1 -> Bus Creator74/17  "HdrstFrwdBkwdnwdPosMax"
  PA_KeSMSw4sLyingMDSecRwRtStHdrstFrwdBkwdnwdPosMin_Val/1 -> Bus Creator74/18  "HdrstFrwdBkwdnwdPosMin"
  PA_KeSMSw4sRecoveryMDSecRwRtStHdrstFrwdBkwdPos_Val/1 -> Bus Creator76/16  "HdrstFrwdBkwdnwdPos"
  PA_KeSMSw4sRecoveryMDSecRwRtStHdrstFrwdBkwdPosMax_Val/1 -> Bus Creator76/17  "HdrstFrwdBkwdnwdPosMax"
  PA_KeSMSw4sRecoveryMDSecRwRtStHdrstFrwdBkwdPosMin_Val/1 -> Bus Creator76/18  "HdrstFrwdBkwdnwdPosMin"
  PA_KeSMSw4sVIPMDSecRwRtStHdrstFrwdBkwdPos_Val/1 -> Bus Creator78/16  "HdrstFrwdBkwdnwdPos"
  PA_KeSMSw4sVIPMDSecRwRtStHdrstFrwdBkwdPosMax_Val/1 -> Bus Creator78/17  "HdrstFrwdBkwdnwdPosMax"
  PA_KeSMSw4sVIPMDSecRwRtStHdrstFrwdBkwdPosMin_Val/1 -> Bus Creator78/18  "HdrstFrwdBkwdnwdPosMin"
  PA_KeSMSwDltTrgtPos_Val241/1 -> Bus Creator53/2  "BkReclnUpwdDnwdPosMax"
  Bus Creator53/1 -> Bus Creator25/6  "FamlyRThdRwRtSt"
  PA_KeSMSwFamilyRMdThdRwRtStFrwdBkwdPos_Val/1 -> Bus Creator53/7  "FrwdBkwdPos"
  PA_KeSMSwDltTrgtPos_Val245/1 -> Bus Creator53/4  "CshnFldUpwdDnwdPos"
  PA_KeSMSwFamilyRMdThdRwRtStFrwdBkwdPosMax_Val/1 -> Bus Creator53/8  "FrwdBkwdPosMax"
  PA_KeSMSwDltTrgtPos_Val243/1 -> Bus Creator53/3  "BkReclnUpwdDnwdPosMin"
  PA_KeSMSwDltTrgtPos_Val244/1 -> Bus Creator53/5  "CshnFldUpwdDnwdPosMax"
  PA_KeSMSwDltTrgtPos_Val242/1 -> Bus Creator53/1  "BkReclnUpwdDnwdPos"
  PA_KeSMSwFamilyRMdThdRwRtStFrwdBkwdPosMin_Val/1 -> Bus Creator53/9  "FrwdBkwdPosMin"
  PA_KeSMSwDltTrgtPos_Val246/1 -> Bus Creator53/6  "CshnFldUpwdDnwdPosMin"
  PA_KeSMSwFamilyLMdThdRwLtStFrwdBkwdPos_Val/1 -> Bus Creator54/7  "FrwdBkwdPos"
  Bus Creator54/1 -> Bus Creator19/6  "FamlyLThdRwLtSt"
  PA_KeSMSwDltTrgtPos_Val251/1 -> Bus Creator54/4  "CshnFldUpwdDnwdPos"
  PA_KeSMSwDltTrgtPos_Val252/1 -> Bus Creator54/6  "CshnFldUpwdDnwdPosMin"
  PA_KeSMSwFamilyLMdThdRwLtStFrwdBkwdPosMax_Val/1 -> Bus Creator54/8  "FrwdBkwdPosMax"
  PA_KeSMSwDltTrgtPos_Val249/1 -> Bus Creator54/3  "BkReclnUpwdDnwdPosMin"
  PA_KeSMSwFamilyLMdThdRwLtStFrwdBkwdPosMin_Val/1 -> Bus Creator54/9  "FrwdBkwdPosMin"
  PA_KeSMSwDltTrgtPos_Val247/1 -> Bus Creator54/2  "BkReclnUpwdDnwdPosMax"
  PA_KeSMSwDltTrgtPos_Val250/1 -> Bus Creator54/5  "CshnFldUpwdDnwdPosMax"
  PA_KeSMSwDltTrgtPos_Val248/1 -> Bus Creator54/1  "BkReclnUpwdDnwdPos"
  PA_KeSMSw6sFamilyLMdThdRwLtStFrwdBkwdPos_Val/1 -> Bus Creator55/7  "FrwdBkwdPos"
  PA_KeSMSwDltTrgtPos_Val98/1 -> Bus Creator55/1  "BkReclnUpwdDnwdPos"
  PA_KeSMSw6sFamilyLMdThdRwLtStFrwdBkwdPosMax_Val/1 -> Bus Creator55/8  "FrwdBkwdPosMax"
  PA_KeSMSwDltTrgtPos_Val113/1 -> Bus Creator55/4  "CshnFldUpwdDnwdPos"
  PA_KeSMSwDltTrgtPos_Val112/1 -> Bus Creator55/5  "CshnFldUpwdDnwdPosMax"
  Bus Creator55/1 -> Bus Creator47/6  "FamlyLThdRwLtSt"
  PA_KeSMSwDltTrgtPos_Val99/1 -> Bus Creator55/3  "BkReclnUpwdDnwdPosMin"
  PA_KeSMSwDltTrgtPos_Val97/1 -> Bus Creator55/2  "BkReclnUpwdDnwdPosMax"
  PA_KeSMSw6sFamilyLMdThdRwLtStFrwdBkwdPosMin_Val/1 -> Bus Creator55/9  "FrwdBkwdPosMin"
  PA_KeSMSwDltTrgtPos_Val114/1 -> Bus Creator55/6  "CshnFldUpwdDnwdPosMin"
  PA_KeSMSwDltTrgtPos_Val255/1 -> Bus Creator56/3  "BkReclnUpwdDnwdPosMin"
  PA_KeSMSw6sFamilyRMdThdRwRtStFrwdBkwdPos_Val/1 -> Bus Creator56/7  "FrwdBkwdPos"
  PA_KeSMSwDltTrgtPos_Val254/1 -> Bus Creator56/1  "BkReclnUpwdDnwdPos"
  PA_KeSMSw6sFamilyRMdThdRwRtStFrwdBkwdPosMin_Val/1 -> Bus Creator56/9  "FrwdBkwdPosMin"
  PA_KeSMSwDltTrgtPos_Val253/1 -> Bus Creator56/2  "BkReclnUpwdDnwdPosMax"
  PA_KeSMSwDltTrgtPos_Val257/1 -> Bus Creator56/4  "CshnFldUpwdDnwdPos"
  Bus Creator56/1 -> Bus Creator52/6  "FamlyRThdRwRtSt"
  PA_KeSMSwDltTrgtPos_Val256/1 -> Bus Creator56/5  "CshnFldUpwdDnwdPosMax"
  PA_KeSMSwDltTrgtPos_Val258/1 -> Bus Creator56/6  "CshnFldUpwdDnwdPosMin"
  PA_KeSMSw6sFamilyRMdThdRwRtStFrwdBkwdPosMax_Val/1 -> Bus Creator56/8  "FrwdBkwdPosMax"
  PA_KeSMSwDltTrgtPos_Val262/1 -> Bus Creator57/5  "BkReclnUpwdDnwdPosMax"
  PA_KeSMSwDltTrgtPos_Val265/1 -> Bus Creator57/11  "HdrstUpwdPosMax"
  PA_KeSMSwDltTrgtPos_Val269/1 -> Bus Creator57/13  "LgrstUpwdPos"
  PA_KeSMSwDltTrgtPos_Val266/1 -> Bus Creator57/10  "HdrstUpwdPos"
  PA_KeSMSwDltTrgtPos_Val263/1 -> Bus Creator57/4  "BkReclnUpwdDnwdPos"
  PA_KeSMSw6sIntimacyRMdSecRwLtStLtwdRtwdPosMax_Val/1 -> Bus Creator57/17  "LtwdRtwdPosMax"
  PA_KeSMSw6sIntimacyRMdSecRwLtStLtwdRtwdPos_Val/1 -> Bus Creator57/16  "LtwdRtwdPos"
  PA_KeSMSwDltTrgtPos_Val268/1 -> Bus Creator57/14  "LgrstUpwdPosMax"
  PA_KeSMSwDltTrgtPos_Val264/1 -> Bus Creator57/6  "BkReclnUpwdDnwdPosMin"
  PA_KeSMSwDltTrgtPos_Val259/1 -> Bus Creator57/2  "ArmScrnPosMax"
  PA_KeSMSwDltTrgtPos_Val270/1 -> Bus Creator57/15  "LgrstUpwdPosMin"
  PA_KeSMSw6sIntimacyRMdSecRwLtStLtwdRtwdPosMin_Val/1 -> Bus Creator57/18  "LtwdRtwdPosMin"
  PA_KeSMSwDltTrgtPos_Val271/1 -> Bus Creator57/8  "FrwdBkwdPosMax"
  PA_KeSMSwDltTrgtPos_Val260/1 -> Bus Creator57/1  "ArmScrnPos"
  PA_KeSMSwDltTrgtPos_Val267/1 -> Bus Creator57/12  "HdrstUpwdPosMin"
  PA_KeSMSwDltTrgtPos_Val272/1 -> Bus Creator57/9  "FrwdBkwdPosMin"
  Bus Creator57/1 -> Bus Creator37/8  "INTMRSecRwLtSt"
  PA_KeSMSwDltTrgtPos_Val261/1 -> Bus Creator57/3  "ArmScrnPosMin"
  PA_KeSMSwDltTrgtPos_Val273/1 -> Bus Creator57/7  "FrwdBkwdPos"
  PA_KeSMSwDltTrgtPos_Val280/1 -> Bus Creator58/5  "BkReclnUpwdDnwdPosMax"
  PA_KeSMSwDltTrgtPos_Val278/1 -> Bus Creator58/1  "ArmScrnPos"
  PA_KeSMSwDltTrgtPos_Val285/1 -> Bus Creator58/12  "HdrstUpwdPosMin"
  PA_KeSMSwDltTrgtPos_Val284/1 -> Bus Creator58/10  "HdrstUpwdPos"
  Bus Creator58/1 -> Bus Creator42/8  "INTMRSecRwRtSt"
  PA_KeSMSw6sIntimacyRMdSecRwRtStLtwdRtwdPosMax_Val/1 -> Bus Creator58/17  "LtwdRtwdPosMax"
  PA_KeSMSwDltTrgtPos_Val282/1 -> Bus Creator58/6  "BkReclnUpwdDnwdPosMin"
  PA_KeSMSwDltTrgtPos_Val286/1 -> Bus Creator58/14  "LgrstUpwdPosMax"
  PA_KeSMSwDltTrgtPos_Val283/1 -> Bus Creator58/11  "HdrstUpwdPosMax"
  PA_KeSMSwDltTrgtPos_Val274/1 -> Bus Creator58/7  "FrwdBkwdPos"
  PA_KeSMSwDltTrgtPos_Val275/1 -> Bus Creator58/9  "FrwdBkwdPosMin"
  PA_KeSMSwDltTrgtPos_Val279/1 -> Bus Creator58/3  "ArmScrnPosMin"
  PA_KeSMSwDltTrgtPos_Val276/1 -> Bus Creator58/8  "FrwdBkwdPosMax"
  PA_KeSMSw6sIntimacyRMdSecRwRtStLtwdRtwdPos_Val/1 -> Bus Creator58/16  "LtwdRtwdPos"
  PA_KeSMSwDltTrgtPos_Val281/1 -> Bus Creator58/4  "BkReclnUpwdDnwdPos"
  PA_KeSMSwDltTrgtPos_Val277/1 -> Bus Creator58/2  "ArmScrnPosMax"
  PA_KeSMSwDltTrgtPos_Val287/1 -> Bus Creator58/13  "LgrstUpwdPos"
  PA_KeSMSwDltTrgtPos_Val288/1 -> Bus Creator58/15  "LgrstUpwdPosMin"
  PA_KeSMSw6sIntimacyRMdSecRwRtStLtwdRtwdPosMin_Val/1 -> Bus Creator58/18  "LtwdRtwdPosMin"
  PA_KeSMSwDltTrgtPos_Val301/1 -> Bus Creator59/7  "FrwdBkwdPos"
  PA_KeSMSwDltTrgtPos_Val302/1 -> Bus Creator59/8  "FrwdBkwdPosMax"
  PA_KeSMSwDltTrgtPos_Val303/1 -> Bus Creator59/9  "FrwdBkwdPosMin"
  PA_KeSMSwDltTrgtPos_Val296/1 -> Bus Creator59/10  "HdrstUpwdPos"
  PA_KeSMSwIntimacyRMdSecRwLtStLtwdRtwdPos_Val/1 -> Bus Creator59/16  "LtwdRtwdPos"
  PA_KeSMSwDltTrgtPos_Val298/1 -> Bus Creator59/14  "LgrstUpwdPosMax"
  PA_KeSMSwIntimacyRMdSecRwLtStLtwdRtwdPosMax_Val/1 -> Bus Creator59/17  "LtwdRtwdPosMax"
  PA_KeSMSwDltTrgtPos_Val300/1 -> Bus Creator59/15  "LgrstUpwdPosMin"
  PA_KeSMSwDltTrgtPos_Val308/1 -> Bus Creator59/4  "BkReclnUpwdDnwdPos"
  PA_KeSMSwDltTrgtPos_Val304/1 -> Bus Creator59/2  "ArmScrnPosMax"
  PA_KeSMSwDltTrgtPos_Val306/1 -> Bus Creator59/3  "ArmScrnPosMin"
  PA_KeSMSwDltTrgtPos_Val305/1 -> Bus Creator59/1  "ArmScrnPos"
  PA_KeSMSwDltTrgtPos_Val295/1 -> Bus Creator59/11  "HdrstUpwdPosMax"
  PA_KeSMSwIntimacyRMdSecRwLtStLtwdRtwdPosMin_Val/1 -> Bus Creator59/18  "LtwdRtwdPosMin"
  PA_KeSMSwDltTrgtPos_Val307/1 -> Bus Creator59/5  "BkReclnUpwdDnwdPosMax"
  Bus Creator59/1 -> Bus Creator14/8  "INTMRSecRwLtSt"
  PA_KeSMSwDltTrgtPos_Val297/1 -> Bus Creator59/12  "HdrstUpwdPosMin"
  PA_KeSMSwDltTrgtPos_Val309/1 -> Bus Creator59/6  "BkReclnUpwdDnwdPosMin"
  PA_KeSMSwDltTrgtPos_Val299/1 -> Bus Creator59/13  "LgrstUpwdPos"
  PA_KeSMSwDltTrgtPos_Val324/1 -> Bus Creator60/7  "FrwdBkwdPos"
  PA_KeSMSwDltTrgtPos_Val322/1 -> Bus Creator60/9  "FrwdBkwdPosMin"
  PA_KeSMSwIntimacyRMdSecRwRtStLtwdRtwdPosMax_Val/1 -> Bus Creator60/17  "LtwdRtwdPosMax"
  PA_KeSMSwDltTrgtPos_Val320/1 -> Bus Creator60/13  "LgrstUpwdPos"
  PA_KeSMSwDltTrgtPos_Val311/1 -> Bus Creator60/1  "ArmScrnPos"
  PA_KeSMSwIntimacyRMdSecRwRtStLtwdRtwdPos_Val/1 -> Bus Creator60/16  "LtwdRtwdPos"
  PA_KeSMSwDltTrgtPos_Val321/1 -> Bus Creator60/15  "LgrstUpwdPosMin"
  PA_KeSMSwDltTrgtPos_Val312/1 -> Bus Creator60/3  "ArmScrnPosMin"
  PA_KeSMSwDltTrgtPos_Val313/1 -> Bus Creator60/5  "BkReclnUpwdDnwdPosMax"
  PA_KeSMSwDltTrgtPos_Val318/1 -> Bus Creator60/12  "HdrstUpwdPosMin"
  PA_KeSMSwDltTrgtPos_Val317/1 -> Bus Creator60/10  "HdrstUpwdPos"
  PA_KeSMSwDltTrgtPos_Val310/1 -> Bus Creator60/2  "ArmScrnPosMax"
  PA_KeSMSwIntimacyRMdSecRwRtStLtwdRtwdPosMin_Val/1 -> Bus Creator60/18  "LtwdRtwdPosMin"
  Bus Creator60/1 -> Bus Creator15/8  "INTMRSecRwRtSt"
  PA_KeSMSwDltTrgtPos_Val314/1 -> Bus Creator60/4  "BkReclnUpwdDnwdPos"
  PA_KeSMSwDltTrgtPos_Val316/1 -> Bus Creator60/11  "HdrstUpwdPosMax"
  PA_KeSMSwDltTrgtPos_Val315/1 -> Bus Creator60/6  "BkReclnUpwdDnwdPosMin"
  PA_KeSMSwDltTrgtPos_Val323/1 -> Bus Creator60/8  "FrwdBkwdPosMax"
  PA_KeSMSwDltTrgtPos_Val319/1 -> Bus Creator60/14  "LgrstUpwdPosMax"
  PA_KeSMSwDltTrgtPos_Val333/1 -> Bus Creator61/18  "HdrstFrwdBkwdnwdPosMin"
  PA_KeSMSwDltTrgtPos_Val332/1 -> Bus Creator61/17  "HdrstFrwdBkwdnwdPosMax"
  PA_KeSMSwDltTrgtPos_Val331/1 -> Bus Creator61/16  "HdrstFrwdBkwdnwdPos"
  Bus Creator61/1 -> Bus Creator79/4  "LgrstOpenLSecRwLtSt"
  PA_KeSMSw4SLegrstOpenMdSecRwLtStFtrstUpwdDnwdPos_Val/1 -> Bus Creator61/13  "FtrstUpwdDnwdPos"
  PA_KeSMSw4SLegrstOpenMdSecRwLtStFtrstUpwdDnwdPosMin_Val/1 -> Bus Creator61/15  "FtrstUpwdDnwdPosMin"
  PA_KeSMSw4SLegrstOpenMdSecRwLtStFtrstUpwdDnwdPosMax_Val/1 -> Bus Creator61/14  "FtrstUpwdDnwdPosMax"
  PA_KeSMSw4SLegrstOpenMdSecRwLtStLgrstOtwdInwdPos_Val/1 -> Bus Creator61/10  "LgrstOtwdInwdPos"
  PA_KeSMSw4SLegrstOpenMdSecRwLtStLgrstOtwdInwdPosMin_Val/1 -> Bus Creator61/12  "LgrstOtwdInwdPosMin"
  PA_KeSMSw4SLegrstOpenMdSecRwLtStLgrstOtwdInwdPosMax_Val/1 -> Bus Creator61/11  "LgrstOtwdInwdPosMax"
  PA_KeSMSw4SLegrstOpenMdSecRwLtStLgrstUpwdDnwdPosMin_Val/1 -> Bus Creator61/9  "LgrstUpwdPosMin"
  PA_KeSMSwDltTrgtPos_Val329/1 -> Bus Creator61/5  "HdrstUpwdPosMax"
  PA_KeSMSwDltTrgtPos_Val326/1 -> Bus Creator61/2  "BkReclnUpwdDnwdPosMax"
  PA_KeSMSwDltTrgtPos_Val328/1 -> Bus Creator61/4  "HdrstUpwdPos"
  PA_KeSMSw4SLegrstOpenMdSecRwLtStLgrstUpwdDnwdPosMax_Val/1 -> Bus Creator61/8  "LgrstUpwdPosMax"
  PA_KeSMSw4SLegrstOpenMdSecRwLtStLgrstUpwdDnwdPos_Val/1 -> Bus Creator61/7  "LgrstUpwdPos"
  PA_KeSMSwDltTrgtPos_Val330/1 -> Bus Creator61/6  "HdrstUpwdPosMin"
  PA_KeSMSwDltTrgtPos_Val327/1 -> Bus Creator61/3  "BkReclnUpwdDnwdPosMin"
  PA_KeSMSwDltTrgtPos_Val336/1 -> Bus Creator62/3  "BkReclnUpwdDnwdPosMin"
  PA_KeSMSwDltTrgtPos_Val339/1 -> Bus Creator62/6  "HdrstUpwdPosMin"
  PA_KeSMSw4SLegrstCloseMdSecRwLtStLgrstUpwdDnwdPos_Val/1 -> Bus Creator62/7  "LgrstUpwdPos"
  PA_KeSMSw4SLegrstCloseMdSecRwLtStLgrstUpwdDnwdPosMax_Val/1 -> Bus Creator62/8  "LgrstUpwdPosMax"
  PA_KeSMSwDltTrgtPos_Val337/1 -> Bus Creator62/4  "HdrstUpwdPos"
  PA_KeSMSwDltTrgtPos_Val334/1 -> Bus Creator62/1  "BkReclnUpwdDnwdPos"
  PA_KeSMSwDltTrgtPos_Val335/1 -> Bus Creator62/2  "BkReclnUpwdDnwdPosMax"
  PA_KeSMSwDltTrgtPos_Val338/1 -> Bus Creator62/5  "HdrstUpwdPosMax"
  PA_KeSMSw4SLegrstCloseMdSecRwLtStLgrstUpwdDnwdPosMin_Val/1 -> Bus Creator62/9  "LgrstUpwdPosMin"
  PA_KeSMSw4SLegrstCloseMdSecRwLtStLgrstOtwdInwdPosMax_Val/1 -> Bus Creator62/11  "LgrstOtwdInwdPosMax"
  PA_KeSMSw4SLegrstCloseMdSecRwLtStLgrstOtwdInwdPosMin_Val/1 -> Bus Creator62/12  "LgrstOtwdInwdPosMin"
  PA_KeSMSw4SLegrstCloseMdSecRwLtStLgrstOtwdInwdPos_Val/1 -> Bus Creator62/10  "LgrstOtwdInwdPos"
  PA_KeSMSw4SLegrstCloseMdSecRwLtStFtrstUpwdDnwdPosMax_Val/1 -> Bus Creator62/14  "FtrstUpwdDnwdPosMax"
  PA_KeSMSw4SLegrstCloseMdSecRwLtStFtrstUpwdDnwdPosMin_Val/1 -> Bus Creator62/15  "FtrstUpwdDnwdPosMin"
  PA_KeSMSw4SLegrstCloseMdSecRwLtStFtrstUpwdDnwdPos_Val/1 -> Bus Creator62/13  "FtrstUpwdDnwdPos"
  Bus Creator62/1 -> Bus Creator79/5  "LgrstCloseLSecRwLtSt"
  PA_KeSMSwDltTrgtPos_Val340/1 -> Bus Creator62/16  "HdrstFrwdBkwdnwdPos"
  PA_KeSMSwDltTrgtPos_Val341/1 -> Bus Creator62/17  "HdrstFrwdBkwdnwdPosMax"
  PA_KeSMSwDltTrgtPos_Val342/1 -> Bus Creator62/18  "HdrstFrwdBkwdnwdPosMin"
  PA_KeSMSwDltTrgtPos_Val351/1 -> Bus Creator65/18  "HdrstFrwdBkwdnwdPosMin"
  PA_KeSMSwDltTrgtPos_Val350/1 -> Bus Creator65/17  "HdrstFrwdBkwdnwdPosMax"
  PA_KeSMSwDltTrgtPos_Val349/1 -> Bus Creator65/16  "HdrstFrwdBkwdnwdPos"
  Bus Creator65/1 -> Bus Creator80/4  "LgrstOpenRSecRwRtSt"
  PA_KeSMSw4SLegrstOpenMdSecRwRtStFtrstUpwdDnwdPos_Val/1 -> Bus Creator65/13  "FtrstUpwdDnwdPos"
  PA_KeSMSwDltTrgtPos_Val347/1 -> Bus Creator65/5  "HdrstUpwdPosMax"
  PA_KeSMSwDltTrgtPos_Val346/1 -> Bus Creator65/4  "HdrstUpwdPos"
  PA_KeSMSwDltTrgtPos_Val343/1 -> Bus Creator65/1  "BkReclnUpwdDnwdPos"
  PA_KeSMSw4SLegrstOpenMdSecRwRtStFtrstUpwdDnwdPosMin_Val/1 -> Bus Creator65/15  "FtrstUpwdDnwdPosMin"
  PA_KeSMSw4SLegrstOpenMdSecRwRtStFtrstUpwdDnwdPosMax_Val/1 -> Bus Creator65/14  "FtrstUpwdDnwdPosMax"
  PA_KeSMSwDltTrgtPos_Val348/1 -> Bus Creator65/6  "HdrstUpwdPosMin"
  PA_KeSMSw4SLegrstOpenMdSecRwRtStLgrstUpwdDnwdPosMax_Val/1 -> Bus Creator65/8  "LgrstUpwdPosMax"
  PA_KeSMSw4SLegrstOpenMdSecRwRtStLgrstUpwdDnwdPosMin_Val/1 -> Bus Creator65/9  "LgrstUpwdPosMin"
  PA_KeSMSwDltTrgtPos_Val344/1 -> Bus Creator65/2  "BkReclnUpwdDnwdPosMax"
  PA_KeSMSw4SLegrstOpenMdSecRwRtStLgrstOtwdInwdPosMax_Val/1 -> Bus Creator65/11  "LgrstOtwdInwdPosMax"
  PA_KeSMSwDltTrgtPos_Val345/1 -> Bus Creator65/3  "BkReclnUpwdDnwdPosMin"
  PA_KeSMSw4SLegrstOpenMdSecRwRtStLgrstOtwdInwdPosMin_Val/1 -> Bus Creator65/12  "LgrstOtwdInwdPosMin"
  PA_KeSMSw4SLegrstOpenMdSecRwRtStLgrstOtwdInwdPos_Val/1 -> Bus Creator65/10  "LgrstOtwdInwdPos"
  PA_KeSMSw4SLegrstOpenMdSecRwRtStLgrstUpwdDnwdPos_Val/1 -> Bus Creator65/7  "LgrstUpwdPos"
  PA_KeSMSw4SLegrstCloseMdSecRwRtStLgrstUpwdDnwdPos_Val/1 -> Bus Creator66/7  "LgrstUpwdPos"
  PA_KeSMSw4SLegrstCloseMdSecRwRtStLgrstOtwdInwdPos_Val/1 -> Bus Creator66/10  "LgrstOtwdInwdPos"
  PA_KeSMSw4SLegrstCloseMdSecRwRtStLgrstOtwdInwdPosMin_Val/1 -> Bus Creator66/12  "LgrstOtwdInwdPosMin"
  PA_KeSMSwDltTrgtPos_Val354/1 -> Bus Creator66/3  "BkReclnUpwdDnwdPosMin"
  PA_KeSMSw4SLegrstCloseMdSecRwRtStLgrstOtwdInwdPosMax_Val/1 -> Bus Creator66/11  "LgrstOtwdInwdPosMax"
  PA_KeSMSwDltTrgtPos_Val353/1 -> Bus Creator66/2  "BkReclnUpwdDnwdPosMax"
  PA_KeSMSw4SLegrstCloseMdSecRwRtStLgrstUpwdDnwdPosMin_Val/1 -> Bus Creator66/9  "LgrstUpwdPosMin"
  PA_KeSMSw4SLegrstCloseMdSecRwRtStLgrstUpwdDnwdPosMax_Val/1 -> Bus Creator66/8  "LgrstUpwdPosMax"
  PA_KeSMSwDltTrgtPos_Val357/1 -> Bus Creator66/6  "HdrstUpwdPosMin"
  PA_KeSMSw4SLegrstCloseMdSecRwRtStFtrstUpwdDnwdPosMax_Val/1 -> Bus Creator66/14  "FtrstUpwdDnwdPosMax"
  PA_KeSMSw4SLegrstCloseMdSecRwRtStFtrstUpwdDnwdPosMin_Val/1 -> Bus Creator66/15  "FtrstUpwdDnwdPosMin"
  PA_KeSMSwDltTrgtPos_Val352/1 -> Bus Creator66/1  "BkReclnUpwdDnwdPos"
  PA_KeSMSwDltTrgtPos_Val355/1 -> Bus Creator66/4  "HdrstUpwdPos"
  PA_KeSMSwDltTrgtPos_Val356/1 -> Bus Creator66/5  "HdrstUpwdPosMax"
  PA_KeSMSw4SLegrstCloseMdSecRwRtStFtrstUpwdDnwdPos_Val/1 -> Bus Creator66/13  "FtrstUpwdDnwdPos"
  Bus Creator66/1 -> Bus Creator80/5  "LgrstCloseRSecRwRtSt"
  PA_KeSMSwDltTrgtPos_Val358/1 -> Bus Creator66/16  "HdrstFrwdBkwdnwdPos"
  PA_KeSMSwDltTrgtPos_Val359/1 -> Bus Creator66/17  "HdrstFrwdBkwdnwdPosMax"
  PA_KeSMSwDltTrgtPos_Val360/1 -> Bus Creator66/18  "HdrstFrwdBkwdnwdPosMin"
  PA_KeSMSwDltTrgtPos_Val325/1 -> Bus Creator61/1  "BkReclnUpwdDnwdPos"
